simulink model "LAB3_2022_finalfinalfinal_real"  (R2022b)
settings: Solver=FixedStepAuto  StartTime=0.0  StopTime=inf  MaxStep=0.1  RelTol=1e-3  EnableMultiTasking=on
PreLoadFcn:
  | % load parameters of the default quadrotor
  | disp('Quadrotor parameters loaded by PreLoadFcn')
  | mdl_quadrotor
values from neighbouring files (symbols this model uses):
  x = [0.0424608327209 0.0421957959129 0.0421507634003 0.0422206614737 0.0422919399693 0.0422554256293 0.0422533212581 0.0423792869681 0.0423405485115 0.0459947200479 0.0487977028194 0.04365098971 ... (480 elements, 480x1)]    [circle_traj.mat]    (also in circle_traj_no_yaw.mat = [0.00634512633233 0.00632005687615 0.00600765127485 0.006498; square_traj.mat = [-0.0634415655034 -0.0633585412536 -0.0633074833692 -0.06343; tilted_circle_traj.mat = [-0.0607553700326 -0.0605675545401 -0.0606748004182 -0.06038)
  y = [3.96225065507 3.96234793823 3.96236175624 3.96233748575 3.96224492439 3.96231073311 3.96229320435 3.96231695889 3.9619596361 3.95424319182 3.95152880377 3.96200027253 ... (480 elements, 480x1)]    [circle_traj.mat]    (also in circle_traj_no_yaw.mat = [4.02713540916 4.02714169293 4.02753378173 4.0271469224 4.02; square_traj.mat = [3.95261374247 3.95279428119 3.95263700747 3.95270560418 3.9; tilted_circle_traj.mat = [4.21432799868 4.2147008566 4.21453844928 4.21462114939 4.21)
  yaw = [-1.57079632679 -1.57079632679 -1.57079632679 -1.57079632679 -1.57079632679 -1.57079632679 -1.57079632679 -1.57079632679 -1.57079632679 -1.57079632679 -1.57079632679 -1.57079632679 ... (480 elements, 480x1)]    [circle_traj.mat]    (also in circle_traj_no_yaw.mat = [-1.57079632679 -1.57079632679 -1.57079632679 -1.57079632679; square_traj.mat = [1.57079632679 1.57079632679 1.57079632679 1.57079632679 1.5; tilted_circle_traj.mat = [-1.57079632679 -1.57079632679 -1.57079632679 -1.57079632679)
  z = [0.108415370891 0.108400378376 0.108421146085 0.108402335438 0.108302960301 0.108325632933 0.108331309827 0.10833915232 0.109410470825 0.186895826135 0.302945157238 0.436490451099 ... (480 elements, 480x1)]    [circle_traj.mat]    (also in circle_traj_no_yaw.mat = [0.107556349257 0.107562483116 0.107663046685 0.107537176932; square_traj.mat = [0.10749365616 0.107370203293 0.107337636345 0.107399519876 ; tilted_circle_traj.mat = [0.107069436595 0.106962311024 0.107025323666 0.107130283357)
undefined symbols (not defined in the file or in its folder): angdiff, Angular, Linear, rot2
libraries: robotlib x4, simulink x1
settings Model: Creator=corkep  LastModifiedBy=crazy1
settings SolverCC: AlgebraicLoopSolver=TrustRegion
settings DataIOCC: LimitDataPoints=on  ReturnWorkspaceOutputs=off
settings OptimizationCC: EnhancedBackFolding=on  PassReuseOutputArgsThreshold=0  ExpressionDepthLimit=2147483647  MaxStackSize=64  OptimizeBlockOrder=speed  DifferentSizesBufferReuse=on  OptimizationCustomize=off
settings DebuggingCC: UnderspecifiedInitializationDetection=Classic  MergeDetectMultiDrivingBlocksExec=none  SolverPrmCheckMsg=warning  ParameterTunabilityLossMsg=error  UnconnectedInputMsg=warning  UnconnectedOutputMsg=warning  UnconnectedLineMsg=warning  AllowSymbolicDim=off  StateNameClashWarn=warning  SFUnexpectedBacktrackingDiag=warning  SFNoUnconditionalDefaultTransitionDiag=warning  SFExecutionAtInitializationDiag=none  ArithmeticOperatorsInVariantConditions=warning
settings HardwareCC: ProdBitPerPointer=32  ProdBitPerSizeT=32  ProdBitPerPtrDiffT=32  ProdLargestAtomicFloat=None  ProdIntDivRoundTo=Undefined  ProdEndianess=Unspecified  ProdWordSize=32  ProdHWDeviceType=Generic->Unspecified (assume 32-bit Generic)  UseEmbeddedCoderFeatures=off
settings ModelReferenceCC: EnableRefExpFcnMdlSchedulingChecks=on  PropagateSignalLabelsOutOfModel=off
settings SFSimCC: SimUseLocalCustomCode=off  MATLABDynamicMemAlloc=off  CustomCodeUndefinedFunction=UseInterfaceOnly
settings RTWCC: Description=Embedded Coder  SystemTargetFile=ert.tlc  HardwareBoard=Robot Operating System (ROS)  TLCOptions="-aInlineSetEventsForThisBaseRateFcn=TLC_FALSE -aSuppressMultiTaskScheduler=TLC_FALSE  -aRateBasedStepFcn=0"  TemplateMakefile=ert_default_tmf  RTWUseLocalCustomCode=off  Toolchain=Catkin  TargetLang=C++  DLArmComputeVersion=19.05
settings CodeAppCC: ForceParamTrailComments=on  OperatorAnnotations=on
settings ERTTargetCC: ERTCustomFileBanners=off  SupportContinuousTime=on  SupportNonInlinedSFcns=on  RemoveResetFunc=off  ModelStepFunctionPrototypeControlCompliant=off
settings ConfigComp: CovMetricSettings=dw  CovSaveCumulativeToWorkspaceVar=on  CovSaveSingleToWorkspaceVar=on  CovExternalEMLEnable=off  CovSFcnEnable=off

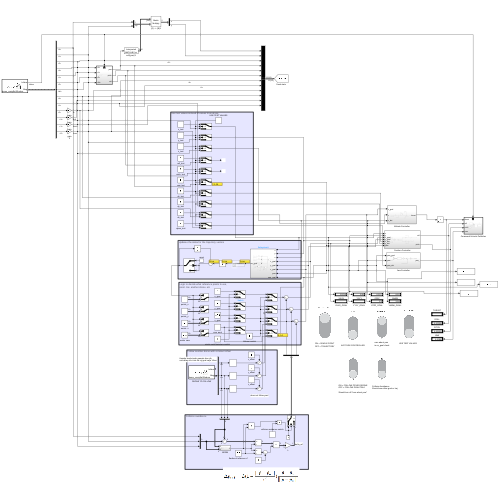
[thumbnail: Simulink's stored preview of the top-level diagram]
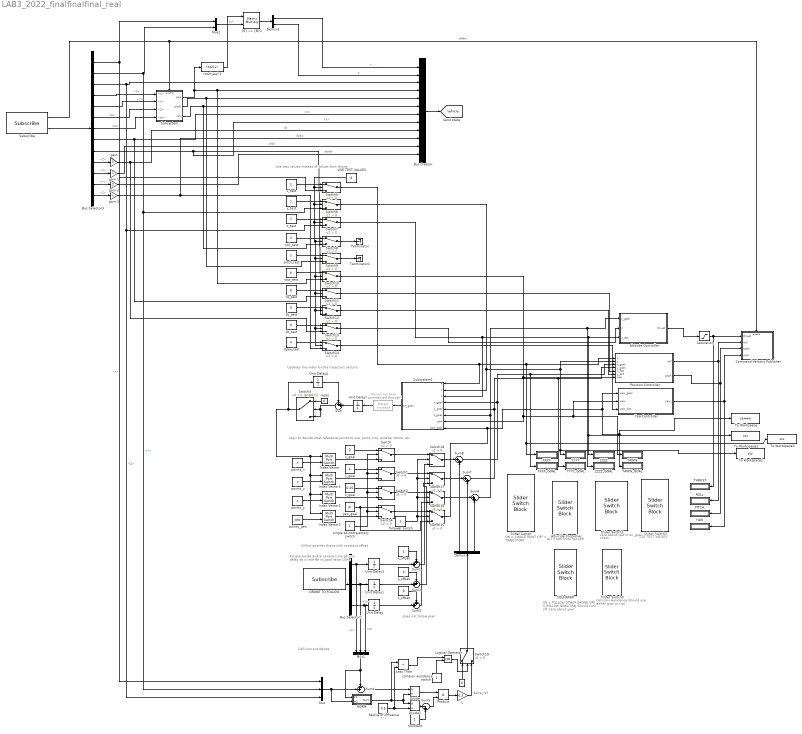
== system LAB3_2022_finalfinalfinal_real ==
  note: Logic to decide what reference points to use,
      | point, traj, another drone, etc
  note: Collision avoidance
  note: delta_ref
  note: Kanske borde ändra sample time på
      | unit delay så vi inte får ny goal varje 10ms
  note: Collision Avoidance
      | Should use either goal or traj
  note: does not follow yaw!
  note: Follow another drone with constant offset
  note: ON = FOLLOW OTHER DRONE
      | OFF = FOLLOW GOAL/TRAJ
      |
      | Should turn off "care about yaw"
  note: Use test values instead of values from drone
  note: USE TEST VALUES
  note: care about yaw
      | in on_goal check
  note: ON = SINGLE POINT
      | OFF = TRAJECTORY
  note: Updates the index for the trajectory vectors
  note: ALTITUDE CONTROLLER
  " " : Constant  Value=0
  Altitude Controller : Subsystem
  Altiutide Controller : SliderSwitchBlock
      settings: Values={{'Off', 'On'}, [0 1]}
  Bus Creator : BusCreator  Inputs=12
  Bus Selector1 : BusSelector  OutputSignals=Pose.Pose.Position.X,Pose.Pose.Position.Y,Pose.Pose.Position.Z
  Bus Selector3 : BusSelector  OutputSignals=Pose.Pose.Position.X,Pose.Pose.Position.Y,Pose.Pose.Position.Z,Pose.Pose.Orientation.X,Pose.Pose.Orientation.Y,Pose.Pose.Orientation.Z,Pose.Pose.Orientation.W,Twist.Twist.Linear.X,Twist.Twist.Linear.Y,Twist.Twist.Linear.Z,Twist.Twist.Angular.X,Twist.Twist.Angular.Y,Twist.Twist.Angular.Z
  Command Velocity Publisher : Subsystem
  Constant : Constant
  DRONE TO FOLLOW : robotlib/Subscribe  topicSource=Select from ROS network  topic=/pixy/vicon/demo_crazyflie28/demo_crazyflie28/odom  messageType=nav_msgs/Odometry  SampleTime=-1  legacyBusStruct=off  messageQueueLength=51
  Demux : Demux  Outputs=3
  Demux1 : Demux  Outputs=2
  Detect Increase : simulink/Logic and Bit Operations/Detect Increase  Commented=through  vinit=0.0  OutDataTypeStr=boolean
  Divide : Product  Inputs=*/
  Divide1 : Product  Inputs=*/
  FOLLOWER : SliderSwitchBlock
      settings: Values={{'Off', 'On'}, [1 0]}
  Index Vector{,1..3} (4 alike) : MultiPortSwitch  DataPortOrder=Zero-based contiguous  Inputs=1  zeroidx=on  SaturateOnIntegerOverflow=off  InputSameDT=off
  L : Gain  Gain=0.3
  Less Than : RelationalOperator  Operator=<  OutDataTypeStr=boolean  RndMeth=Simplest  InputSameDT=off
  Logical Operator : Logic  Operator=OR  AllPortsSameDT=off  OutDataTypeStr=boolean
  Mux : Mux  Inputs=3
  Mux1 : Mux  Inputs=3
  Mux2 : Mux  Inputs=2
  NORM : Subsystem
  PITCH : Display
  Position Controller : Subsystem
  Product : Product
  ROLL : Display
  Radius of influence r^i : Constant  Value=0.5
  Saturation : Saturate  UpperLimit=0.8  LowerLimit=0
  Slider Switch{,1..3} (4 alike) : SliderSwitchBlock
  Subscribe : robotlib/Subscribe  topicSource=Select from ROS network  topic=/pixy/vicon/demo_crazyflie28/demo_crazyflie28/odom  messageType=nav_msgs/Odometry  SampleTime=-1  legacyBusStruct=off  messageQueueLength=51
  Subsystem : Subsystem
  Subsystem1 : Subsystem
  Sum{,1..3} (4 alike) : Sum  Inputs=++|
  Sum4 : Sum  Inputs=-+|
  Sum5 : Sum  Inputs=|-+
  Sum6 : Sum  Inputs=|++
  Sum7 : Sum  Inputs=|++
  Sum8 : Sum  Inputs=|++
  Switch{,1..2,4..19} (19 alike) : Switch  Criteria=u2 > Threshold  SaturateOnIntegerOverflow=off  InputSameDT=off
  Switch3 : Switch  Threshold=length(x)  SaturateOnIntegerOverflow=off  InputSameDT=off
  THRUST : Display
  Terminator : Terminator
  Terminator1 : Terminator
  To Workspace : ToWorkspace  VariableName=yawww  SaveFormat=Timeseries  SampleTime=-1
  To Workspace1 : ToWorkspace  VariableName=zzz  SaveFormat=Timeseries  SampleTime=-1
  To Workspace2 : ToWorkspace  VariableName=yyy  SaveFormat=Timeseries  SampleTime=-1
  To Workspace3 : ToWorkspace  VariableName=xxx  SaveFormat=Timeseries  SampleTime=-1
  USE TEST VALUES : Constant  Value=0
  Unit Delay{,1..4} (5 alike) : UnitDelay  SampleTime=-1  HasFrameUpgradeWarning=on
  XXXX : Display
  XXXX_GOAL : Display
  YAW : Display
  YAWW : Display
  YAWW_GOAL : Display
  YYYY : Display
  YYYY_GOAL : Display
  Yaw Controller : Subsystem
  ZZZZ : Display
  ZZZZ_GOAL : Display
  collision avoidance switch : Constant
  dx_test : Constant  Value=0
  dy_test : Constant  Value=0
  dyaw_test : Constant  Value=0
  dz_test : Constant  Value=0
  follower switch : Constant
  gain {,1..3} (4 alike) : Gain
  pitch_test : Constant
  points_x : Constant  Value=x
  points_y : Constant  Value=y
  points_yaw : Constant  Value=yaw
  points_z : Constant  Value=z
  reset : Constant  Value=0  VectorParams1D=off
  roll_test : Constant
  rot2(yaw)'1 : MATLABFcn  MATLABFcn=rot2(u)'  OutputDimensions=[2 2]  Output1D=off
  single point/trajectory switch : Constant
  x_goal : Constant  Value=0
  x_offset : Constant
  x_test : Constant
  y_goal : Constant  Value=4
  y_offset : Constant  Value=0
  y_test : Constant
  yaw_goal : Constant  Value=pi
  yaw_test : Constant  Value=0
  z_goal : Constant  Value=0.25
  z_offset : Constant  Value=0
  z_test : Constant
  "{0} --> {B}1" : Product  Multiplication=Matrix(*)  RndMeth=Zero
  tag scope: vehicle=global
  wires:
  Bus Selector3/11 -> gain 1/1  "<X>"
  Bus Selector3/13 -> gain 3/1  "<Z>"
  Bus Selector3/10 -> "gain "/1  "<Z>"
  Bus Selector3/9 -> Switch12/3, Bus Creator/8  "<Y>"
  Bus Selector3/8 -> Switch11/3, Bus Creator/7  "<X>"
  Bus Selector3/3 -> Mux/3, Switch7/3, Bus Creator/3  "<Z>"
  Bus Creator/1 -> [vehicle]
  Bus Selector3/12 -> gain 2/1  "<Y>"
  Subscribe/2 -> Bus Selector3/1
  Subscribe/1 -> Subsystem/Enable, Command Velocity Publisher/Enable  "IsNew"
  Mux2/1 -> "{0} --> {B}1"/2  "xy*"
  "{0} --> {B}1"/1 -> Demux1/1
  Demux1/1 -> Bus Creator/1  "x"
  Demux1/2 -> Bus Creator/2  "y"
  Bus Selector3/1 -> Mux/1, Mux2/1, Switch5/3  "<X>"
  Bus Selector3/2 -> Mux/2, Switch6/3, Mux2/2  "<Y>"
  rot2(yaw)'1/1 -> "{0} --> {B}1"/1
  "gain "/1 -> Switch13/3, Bus Creator/9  "dz"
  gain 1/1 -> Bus Creator/11  "droll"
  gain 2/1 -> Bus Creator/12  "dpitch"
  gain 3/1 -> Switch14/3, Bus Creator/10  "dyaw"
  Subsystem/1(yaw) -> rot2(yaw)'1/1, Switch10/3, Bus Creator/4
  Bus Selector3/4 -> Subsystem/1(<X>)  "<X>"
  Bus Selector3/5 -> Subsystem/2(<Y>)  "<Y>"
  Bus Selector3/6 -> Subsystem/3(<Z>)  "<Z>"
  Bus Selector3/7 -> Subsystem/4(<W>)  "<W>"
  Subsystem/2(pitch) -> Switch9/3, Bus Creator/5
  Subsystem/3(roll) -> Switch8/3, Bus Creator/6
  Altitude Controller/1(thrust) -> Saturation/1
  Saturation/1 -> Command Velocity Publisher/1(thrust), THRUST/1
  Position Controller/2(pitch) -> PITCH/1, Command Velocity Publisher/3(pitch)
  Position Controller/1(roll) -> ROLL/1, Command Velocity Publisher/2(roll)
  Yaw Controller/1(yaw_) -> Command Velocity Publisher/4(yaw), YAW/1
  Unit Delay4/1 -> Sum/1
  Sum/1 -> Switch3/3, Switch3/2
  Unit Delay2/1 -> Sum/2
  reset/1 -> Switch3/1
  Detect Increase/1 -> Unit Delay2/1
  Subsystem1/1(on_goal) -> Detect Increase/1
  points_x/1 -> Index Vector/2
  points_y/1 -> Index Vector1/2
  points_z/1 -> Index Vector2/2
  points_yaw/1 -> Index Vector3/2
  Sum8/1 -> Position Controller/3(x_goal), XXXX_GOAL/1, Subsystem1/4(x_goal)
  Index Vector/1 -> Switch/3
  Index Vector1/1 -> Switch1/3
  Index Vector2/1 -> Switch2/3
  Index Vector3/1 -> Switch4/3
  single point/trajectory switch/1 -> Switch/2, Switch1/2, Switch2/2, Switch4/2
  Switch15/1 -> Subsystem1/8(yaw_goal), YAWW_GOAL/1, To Workspace/1, Yaw Controller/1(yaw_goal)
  Sum6/1 -> Altitude Controller/1(z_goal), ZZZZ_GOAL/1, Subsystem1/6(z_goal)
  Sum7/1 -> Position Controller/4(y_goal), YYYY_GOAL/1, Subsystem1/5(y_goal)
  x_test/1 -> Switch5/1
  y_test/1 -> Switch6/1
  z_test/1 -> Switch7/1
  USE TEST VALUES/1 -> Switch14/2, Switch13/2, Switch12/2, Switch11/2, Switch10/2, Switch9/2, Switch8/2, Switch7/2, Switch6/2, Switch5/2
  roll_test/1 -> Switch8/1
  pitch_test/1 -> Switch9/1
  yaw_test/1 -> Switch10/1
  dx_test/1 -> Switch11/1
  dy_test/1 -> Switch12/1
  dz_test/1 -> Switch13/1
  dyaw_test/1 -> Switch14/1
  Switch7/1 -> Subsystem1/3(z), Altitude Controller/2(z), ZZZZ/1, To Workspace1/1
  Switch5/1 -> Position Controller/1(x), To Workspace3/1, XXXX/1, Subsystem1/1(x)
  Switch6/1 -> Position Controller/2(y), To Workspace2/1, YYYY/1, Subsystem1/2(y)
  Switch8/1 -> Terminator/1
  Switch10/1 -> Subsystem1/7(yaw), YAWW/1, Yaw Controller/2(yaw), Position Controller/7(yaw)
  Switch11/1 -> Position Controller/5(x_dot)
  Switch12/1 -> Position Controller/6(y_dot)
  Switch13/1 -> Altitude Controller/3(z_dot)
  Switch14/1 -> Yaw Controller/3(yaw_dot)
  Switch9/1 -> Terminator1/1
  x_goal/1 -> Switch/1
  y_goal/1 -> Switch1/1
  z_goal/1 -> Switch2/1
  yaw_goal/1 -> Switch15/3, Switch4/1
  Switch3/1 -> Index Vector3/1, Index Vector2/1, Index Vector1/1, Index Vector/1, Unit Delay4/1
  Switch/1 -> Switch18/1
  Switch1/1 -> Switch17/1
  Switch2/1 -> Switch16/1
  Switch4/1 -> Switch15/1
  follower switch/1 -> Switch18/2, Switch17/2, Switch16/2, Switch15/2
  DRONE TO FOLLOW/2 -> Bus Selector1/1
  Bus Selector1/3 -> Unit Delay/1, Mux1/3  "<Z>"
  z_offset/1 -> Sum3/1
  Bus Selector1/2 -> Unit Delay1/1, Mux1/2  "<Y>"
  y_offset/1 -> Sum2/1
  Bus Selector1/1 -> Unit Delay3/1, Mux1/1  "<X>"
  x_offset/1 -> Sum1/1
  Sum1/1 -> Switch18/3
  Sum2/1 -> Switch17/3
  Sum3/1 -> Switch16/3
  Unit Delay/1 -> Sum3/2
  Unit Delay1/1 -> Sum2/2
  Unit Delay3/1 -> Sum1/2
  Mux/1 -> Sum4/2, NORM/2(In2)
  Mux1/1 -> NORM/1(In1), Sum4/1
  Sum4/1 -> Divide/1
  NORM/1(Out1) -> Less Than/1, Divide1/1, Divide/2
  Radius of influence r^i/1 -> Less Than/2, Divide1/2
  Constant/1 -> Sum5/2
  Divide/1 -> Product/1
  Divide1/1 -> Sum5/1
  Product/1 -> L/1
  L/1 -> Switch19/3
  collision avoidance switch/1 -> Logical Operator/2
  " "/1 -> Switch19/1
  Switch19/1 -> Demux/1
  Switch16/1 -> Sum6/1
  Switch17/1 -> Sum7/1
  Switch18/1 -> Sum8/1
  Demux/2 -> Sum7/2
  Demux/1 -> Sum8/2
  Demux/3 -> Sum6/2
  Less Than/1 -> Logical Operator/1
  Logical Operator/1 -> Switch19/2
  Sum5/1 -> Product/2

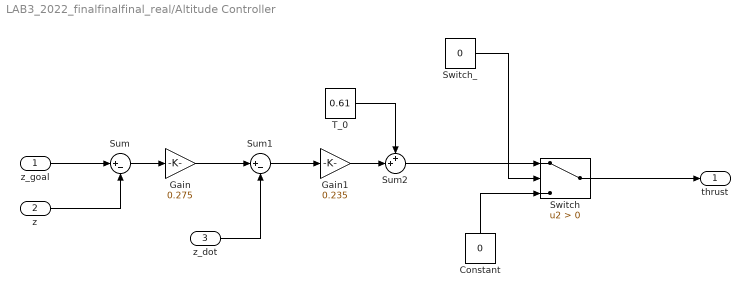
== system LAB3_2022_finalfinalfinal_real/Altitude Controller ==
  z_goal : Inport  PortDimensions=1
  z : Inport  Port=2
  z_dot : Inport  Port=3
  Constant : Constant  Value=0
  Gain : Gain  Gain=0.275
  Gain1 : Gain  Gain=0.235
  Sum : Sum  Inputs=|+-
  Sum1 : Sum  Inputs=|+-
  Sum2 : Sum  Inputs=++|
  Switch : Switch  Criteria=u2 > Threshold  SaturateOnIntegerOverflow=off  InputSameDT=off
  Switch_ : Constant  Value=0
  T_0 : Constant  Value=0.61
  thrust : Outport
  wires:
  z_goal/1 -> Sum/1
  z/1 -> Sum/2
  Sum2/1 -> Switch/1
  Switch/1 -> thrust/1
  Constant/1 -> Switch/3
  Switch_/1 -> Switch/2
  Sum/1 -> Gain/1
  Sum1/1 -> Gain1/1
  T_0/1 -> Sum2/1
  Gain/1 -> Sum1/1
  z_dot/1 -> Sum1/2
  Gain1/1 -> Sum2/2

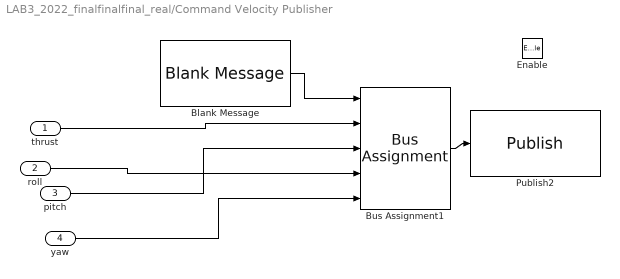
== system LAB3_2022_finalfinalfinal_real/Command Velocity Publisher ==
  thrust : Inport
  roll : Inport  Port=2
  pitch : Inport  Port=3
  yaw : Inport  Port=4
  Enable : EnablePort
  Blank Message : robotlib/Blank Message  messageClass=Message  entityType=geometry_msgs/Twist  messageType=geometry_msgs/Twist  SampleTime=inf  legacyBusStruct=off
  Bus Assignment1 : BusAssignment  DialogController=Simulink.DDGSource_BusAssignment  AssignedSignals=Linear.Z,Linear.X,Linear.Y,Angular.Z
  Publish2 : robotlib/Publish  topicSource=Select from ROS network  topic=/demo_crazyflie28/cmd_vel  messageType=geometry_msgs/Twist  legacyBusStruct=off  messageQueueLength=105
  wires:
  Bus Assignment1/1 -> Publish2/1
  Blank Message/1 -> Bus Assignment1/1
  yaw/1 -> Bus Assignment1/5
  roll/1 -> Bus Assignment1/4
  pitch/1 -> Bus Assignment1/3
  thrust/1 -> Bus Assignment1/2

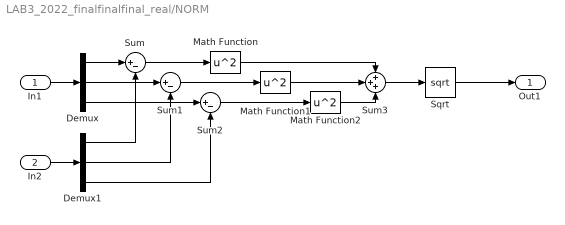
== system LAB3_2022_finalfinalfinal_real/NORM ==
  In1 : Inport
  In2 : Inport  Port=2
  Demux : Demux  Outputs=3
  Demux1 : Demux  Outputs=3
  Math Function : Math  Operator=square
  Math Function1 : Math  Operator=square
  Math Function2 : Math  Operator=square
  Sqrt : Sqrt
  Sum : Sum  Inputs=|+-
  Sum1 : Sum  Inputs=|+-
  Sum2 : Sum  Inputs=|+-
  Sum3 : Sum  Inputs=+++
  Out1 : Outport
  wires:
  In1/1 -> Demux/1
  In2/1 -> Demux1/1
  Demux/3 -> Sum2/1
  Demux/1 -> Sum/1
  Demux/2 -> Sum1/1
  Demux1/1 -> Sum/2
  Demux1/2 -> Sum1/2
  Demux1/3 -> Sum2/2
  Sum/1 -> Math Function/1
  Sum1/1 -> Math Function1/1
  Sum2/1 -> Math Function2/1
  Math Function1/1 -> Sum3/2
  Math Function2/1 -> Sum3/3
  Math Function/1 -> Sum3/1
  Sum3/1 -> Sqrt/1
  Sqrt/1 -> Out1/1

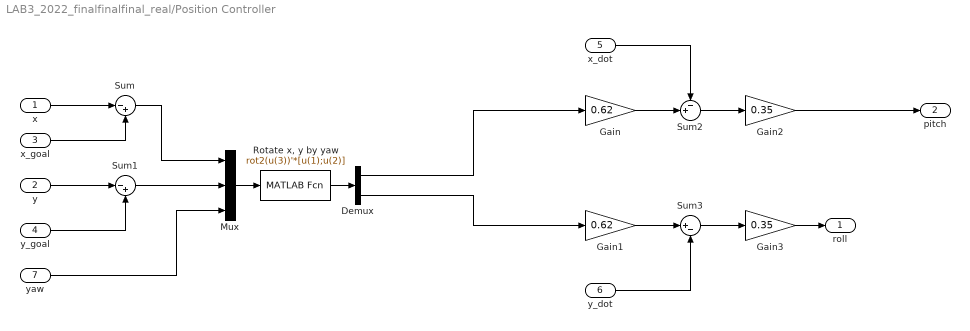
== system LAB3_2022_finalfinalfinal_real/Position Controller ==
  x : Inport
  y : Inport  Port=2
  x_goal : Inport  Port=3  PortDimensions=1
  y_goal : Inport  Port=4  PortDimensions=1
  x_dot : Inport  Port=5
  y_dot : Inport  Port=6
  yaw : Inport  Port=7
  Demux : Demux  Outputs=2
  Gain : Gain  Gain=0.62
  Gain1 : Gain  Gain=0.62
  Gain2 : Gain  Gain=0.35
  Gain3 : Gain  Gain=0.35
  Mux : Mux  Inputs=3
  "Rotate x, y by yaw" : MATLABFcn  MATLABFcn=rot2(u(3))'*[u(1);u(2)]
  Sum : Sum  Inputs=|-+
  Sum1 : Sum  Inputs=|-+
  Sum2 : Sum  Inputs=-+|
  Sum3 : Sum  Inputs=|+-
  roll : Outport
  pitch : Outport  Port=2
  wires:
  y/1 -> Sum1/1
  y_goal/1 -> Sum1/2
  x/1 -> Sum/1
  x_goal/1 -> Sum/2
  Gain1/1 -> Sum3/1
  Gain/1 -> Sum2/2
  Sum3/1 -> Gain3/1
  Sum2/1 -> Gain2/1
  y_dot/1 -> Sum3/2
  x_dot/1 -> Sum2/1
  Mux/1 -> "Rotate x, y by yaw"/1
  Sum/1 -> Mux/1
  Sum1/1 -> Mux/2
  yaw/1 -> Mux/3
  "Rotate x, y by yaw"/1 -> Demux/1
  Demux/1 -> Gain/1
  Demux/2 -> Gain1/1
  Gain3/1 -> roll/1
  Gain2/1 -> pitch/1

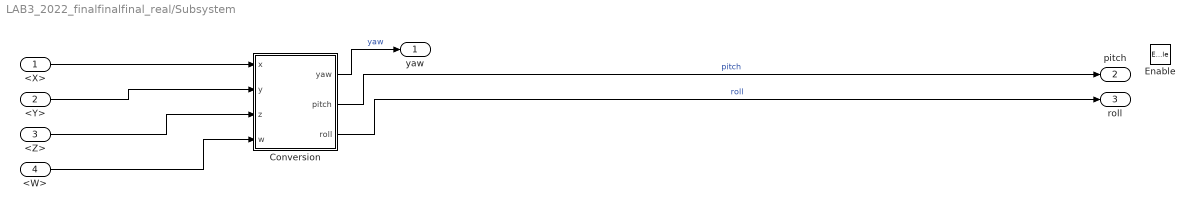
== system LAB3_2022_finalfinalfinal_real/Subsystem ==
  <X> : Inport
  <Y> : Inport  Port=2
  <Z> : Inport  Port=3
  <W> : Inport  Port=4
  Enable : EnablePort
  Conversion : MATLAB Function  TreatAsAtomicUnit=on
  yaw : Outport
  pitch : Outport  Port=2
  roll : Outport  Port=3
  wires:
  Conversion/1(yaw) -> yaw/1  "yaw"
  <X>/1 -> Conversion/1(x)
  Conversion/2(pitch) -> pitch/1  "pitch"
  <W>/1 -> Conversion/4(w)
  <Y>/1 -> Conversion/2(y)
  Conversion/3(roll) -> roll/1  "roll"
  <Z>/1 -> Conversion/3(z)

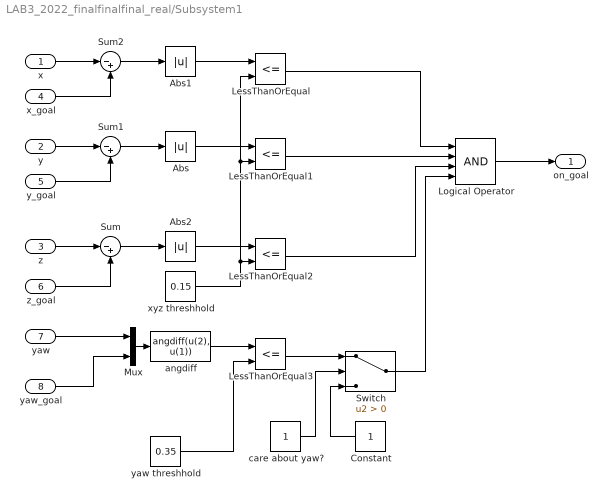
== system LAB3_2022_finalfinalfinal_real/Subsystem1 ==
  x : Inport
  y : Inport  Port=2
  z : Inport  Port=3
  x_goal : Inport  Port=4
  y_goal : Inport  Port=5
  z_goal : Inport  Port=6
  yaw : Inport  Port=7
  yaw_goal : Inport  Port=8  PortDimensions=1
  Abs : Abs  SaturateOnIntegerOverflow=off
  Abs1 : Abs  SaturateOnIntegerOverflow=off
  Abs2 : Abs  SaturateOnIntegerOverflow=off
  Constant : Constant
  LessThanOrEqual{,1..3} (4 alike) : RelationalOperator  Operator=<=  OutDataTypeStr=boolean  RndMeth=Simplest  InputSameDT=off
  Logical Operator : Logic  Inputs=4  AllPortsSameDT=off  OutDataTypeStr=boolean
  Mux : Mux  Inputs=2
  Sum : Sum  Inputs=|-+
  Sum1 : Sum  Inputs=|-+
  Sum2 : Sum  Inputs=|-+
  Switch : Switch  Criteria=u2 > Threshold  SaturateOnIntegerOverflow=off  InputSameDT=off
  angdiff : MATLABFcn  MATLABFcn=angdiff(u(2), u(1))
  care about yaw? : Constant
  xyz threshhold : Constant  Value=0.15
  yaw threshhold : Constant  Value=0.35
  on_goal : Outport
  wires:
  z/1 -> Sum/1
  y/1 -> Sum1/1
  x/1 -> Sum2/1
  x_goal/1 -> Sum2/2
  y_goal/1 -> Sum1/2
  z_goal/1 -> Sum/2
  Sum2/1 -> Abs1/1
  Sum1/1 -> Abs/1
  Sum/1 -> Abs2/1
  Logical Operator/1 -> on_goal/1
  Abs1/1 -> LessThanOrEqual/1
  Abs/1 -> LessThanOrEqual1/1
  Abs2/1 -> LessThanOrEqual2/1
  xyz threshhold/1 -> LessThanOrEqual/2, LessThanOrEqual1/2, LessThanOrEqual2/2
  LessThanOrEqual/1 -> Logical Operator/1
  LessThanOrEqual1/1 -> Logical Operator/2
  LessThanOrEqual2/1 -> Logical Operator/3
  Mux/1 -> angdiff/1
  angdiff/1 -> LessThanOrEqual3/1
  Constant/1 -> Switch/3
  LessThanOrEqual3/1 -> Switch/1
  Switch/1 -> Logical Operator/4
  care about yaw?/1 -> Switch/2
  yaw/1 -> Mux/1
  yaw_goal/1 -> Mux/2
  yaw threshhold/1 -> LessThanOrEqual3/2

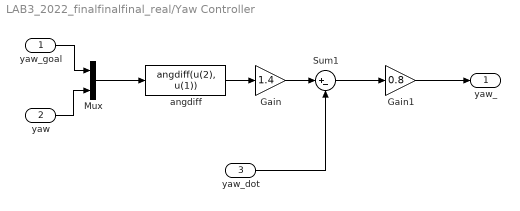
== system LAB3_2022_finalfinalfinal_real/Yaw Controller ==
  yaw_goal : Inport  PortDimensions=1
  yaw : Inport  Port=2
  yaw_dot : Inport  Port=3
  Gain : Gain  Gain=1.4
  Gain1 : Gain  Gain=0.8
  Mux : Mux  Inputs=2
  Sum1 : Sum  Inputs=|+-
  angdiff : MATLABFcn  MATLABFcn=angdiff(u(2), u(1))
  yaw_ : Outport
  wires:
  yaw_goal/1 -> Mux/1
  yaw/1 -> Mux/2
  angdiff/1 -> Gain/1
  Gain/1 -> Sum1/1
  Sum1/1 -> Gain1/1
  yaw_dot/1 -> Sum1/2
  Gain1/1 -> yaw_/1
  Mux/1 -> angdiff/1

== matlab function LAB3_2022_finalfinalfinal_real/Subsystem/Conversion ==
  data: yaw output; x input; y input; z input; w input; pitch output; roll output
function [yaw,pitch,roll]  = quat2eul(x,y,z,w)
%#codegen

% Convert the quaternion to a yaw angle (zyx euler angle)
eul = quat2eul([w,x,y,z]);
yaw = eul(1);
roll = eul(3);
pitch = eul(2);

end
